simulink model "Simulador_Telemetria"  (R2015a)
settings: Solver=ode45  StartTime=0.0  StopTime=entrada2  RelTol=1e-6  AbsTol=1e-6
StopFcn:
  | close all;
  | post_simulacion_telemetria;
model workspace (MAT data in the model file):
  m = 3.797
  b = 2.1
  c = 0.3571
  Salar = 0.75
  AR = 5.88
  cg = [0.44 0 0]
  Ix = 1.229
  Iy = 0.1702
  Iz = 0.8808
  Ixz = 0.9343
  e = 0.9935
  alpha0 = 0.267
  coefprop = [0.016415 -0.0142726]
  C_L0 = 0.0254
  C_Lalpha = 4.0191
  C_Lq = 3.8954
  C_Ldelta_e = 0.5872
  C_D0 = 0.0102
  C_Dbeta1 = -2.0864e-07
  C_Dbeta2 = 0.0671
  C_Dq = 0
  C_Ddelta_e = 0.8461
  C_Y0 = 3.2049e-18
  C_Ybeta = -0.1949
  C_Yp = -0.1172
  C_Yr = 0.0959
  C_Ydelta_a = -0.0696
  C_l0 = 1.1518e-18
  C_lbeta = -0.0765
  C_lp = -0.4018
  C_lr = 0.025
  C_ldelta_a = 0.2987
  C_m0 = 0.018
  C_malpha = -0.2524
  C_mq = -1.3047
  C_mdelta_e = -0.4857
  C_n0 = -2.2667e-07
  C_nbeta = 0.0403
  C_np = -0.0247
  C_nr = -0.1252
  C_ndelta_a = 0.0076
  gamma = 0.20958671
  gamma1 = 8.64638926772
  gamma2 = 7.15127867602
  gamma3 = 4.20255654569
  gamma4 = 4.4578208227
  gamma5 = -2.04582843713
  gamma6 = 5.48942420682
  gamma7 = 10.3736620037
  gamma8 = 5.86392142899
  C_p0 = -1.01045424588e-06
  C_pbeta = -0.14184539659
  C_pp = -1.79869539438
  C_pr = -0.45305525336
  C_pdelta_a = 1.28918307845
  C_r0 = -1.3291750703e-06
  C_rbeta = -0.104707259349
  C_rp = -1.93599126586
  C_rr = -0.622717442342
  C_rdelta_a = 1.3761168826
  C_mp = -0.2168
undefined symbols (not defined in the file or in its folder): magnitude
libraries: aerolibconvert2 x9, aerolibfltsims x2, instrumentlib x1, aerolibatmos2 x1, aerolibgravity2 x1
settings Model: TunableVars=GNSS,Viento  TunableVarsStorageClass=Auto,Auto  TunableVarsTypeQualifier=,  Creator=Cecilia Ruiz Romero  LastModifiedBy=Cecilia Ruiz Romero
settings SolverCC: ZeroCrossControl=EnableAll
settings DataIOCC: ExternalInput=[t,u]  SaveOutput=off  TimeSaveName=tiempos

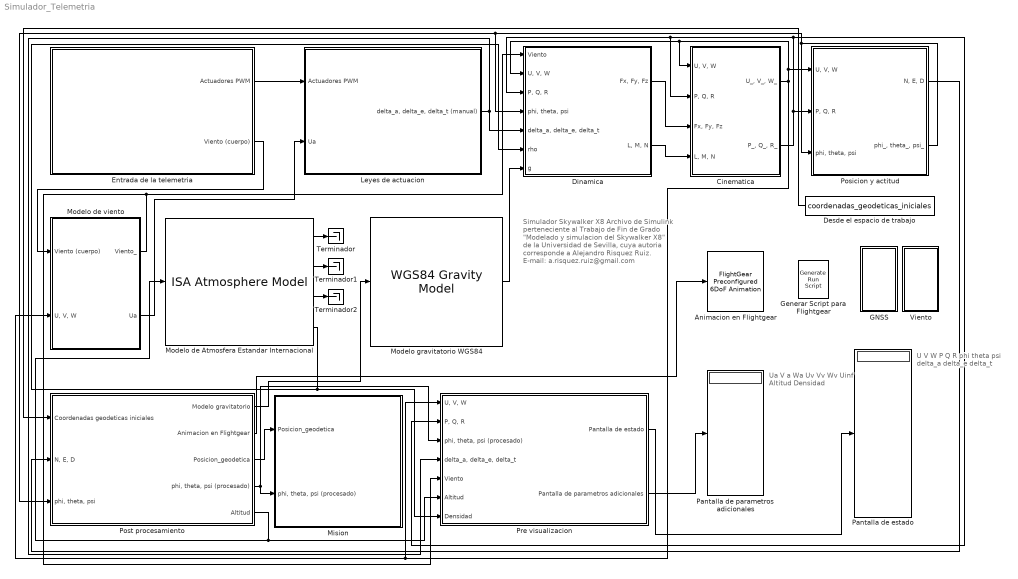
== system Simulador_Telemetria ==
  note: U
      | V
      | W
      | P
      | Q
      | R
      | phi
      | theta
      | psi
      | delta_a
      | delta_e
      | delta_t
  note: Ua
      | V a
      | Wa
      | Uv
      | Vv
      | Wv
      | Uinf
      | Altitud
      | Densidad
  note: Simulador Skywalker X8
      |
      | Archivo de Simulink perteneciente al Trabajo de Fin de Grado "Modelado y simulacion del Skywalker X8" de la Universidad de Sevilla, cuya autoria corresponde a Alejandro Risquez Ruiz.
      |
      | E-mail: a.risquez.ruiz@gmail.com
  Animacion en Flightgear : aerolibfltsims/FlightGear Preconfigured 6DoF Animation  xFlightGearVersion=v3.0  DestinationIpAddress=192.168.1.33  DestinationPort=5502  SampleTime=1/30
  Cinematica : Subsystem
  Desde el espacio de trabajo : FromWorkspace  VariableName=coordenadas_geodeticas_iniciales
  Dinamica : Subsystem
  Entrada de la telemetria : Subsystem
  GNSS : Subsystem  DialogController=hmiCreateDDGDialog  IsWebBlock=on  mask(MathWorksWebBlock){webBlockId=2f82c36a-ef1f-4a61-96ee-8f2028b7861b, webBlockType=toggleswitch, ShowInLibBrowser=on, ShowInitialText=on, HMISrcModelName=Simulador_Telemetria}
      mask prompts: webBlockId "WebBlock Id"; webBlockType "WebBlock Type"; HMISrcModelName "Source Model"
      mask Help: helpview([docroot '/mapfiles/simulink.map'], 'hmi_toggle_switch')
      mask Display:
      | if strcmp(get_param(bdroot(gcb),'BlockDiagramType'), 'library')
      |     image([(matlabroot) '/toolbox/simulink/hmi/icons/ToggleSwitch.png']);
      | end
  Generar Script para Flightgear : aerolibfltsims/Generate Run Script  OutputFileName=Flightgear_simulador.bat  FlightGearBaseDirectory=C:\Program Files\FlightGear  GeometryModelName=Malolo1  DestinationPort=5502  OriginAddress=192.168.1.34  OriginPort=5505  LocalAddress=192.168.1.35  AirportId=LEZL  RunwayId=27  InitialAltitude=328  InitialHeading=270  OffsetDistance=0  OffsetAzimuth=0  GenerateFile=off  Architecture=Win64  dataFlow=Receive
  Leyes de actuacion : Subsystem
  Mision : Subsystem
  Modelo de Atmosfera Estandar Internacional : aerolibatmos2/ISA Atmosphere Model  custom=off  g=9.80665  gamma=1.4  R=287.0531  L=0.0065  h_trop=11000  h_strat=20000  rho0=1.225  P0=101325  T0=288.15  h0=0
  Modelo de viento : Subsystem
  Modelo gravitatorio WGS84 : aerolibgravity2/WGS84 Gravity Model   model=WGS84 Taylor Series  units=Metric (MKS)  no_atmos=on  precessing=on  jd_loc=off  month=October  day=10  year=2004  no_centrifugal=on  action=Warning
  Pantalla de estado : Display
  Pantalla de parametros adicionales : Display
  Posicion y actitud : Subsystem
  Post procesamiento : Subsystem
  Pre visualizacion : Subsystem
  Terminador : Terminator
  Terminador1 : Terminator
  Terminador2 : Terminator
  Viento : Subsystem  DialogController=hmiCreateDDGDialog  IsWebBlock=on  mask(MathWorksWebBlock){webBlockId=de649073-e8b6-4552-a188-ccf5b7e05afd, webBlockType=toggleswitch, ShowInLibBrowser=on, ShowInitialText=on, HMISrcModelName=Simulador_Telemetria}
      mask prompts: webBlockId "WebBlock Id"; webBlockType "WebBlock Type"; HMISrcModelName "Source Model"
      mask Help: helpview([docroot '/mapfiles/simulink.map'], 'hmi_toggle_switch')
      mask Display:
      | if strcmp(get_param(bdroot(gcb),'BlockDiagramType'), 'library')
      |     image([(matlabroot) '/toolbox/simulink/hmi/icons/ToggleSwitch.png']);
      | end
  wires:
  Modelo de Atmosfera Estandar Internacional/1 -> Terminador/1
  Modelo de Atmosfera Estandar Internacional/2 -> Terminador1/1
  Modelo de Atmosfera Estandar Internacional/3 -> Terminador2/1
  Post procesamiento/5(Altitud) -> Modelo de Atmosfera Estandar Internacional/1, Pre visualizacion/6(Altitud)
  Cinematica/1("U_, V_, W_") -> Modelo de viento/2("U, V, W"), Pre visualizacion/1("U, V, W"), Dinamica/2("U, V, W"), Cinematica/1("U, V, W"), Posicion y actitud/1("U, V, W")
  Modelo de viento/1(Viento_) -> Pre visualizacion/5(Viento), Dinamica/1(Viento)
  Modelo de Atmosfera Estandar Internacional/4 -> Pre visualizacion/7(Densidad), Dinamica/6(rho)
  Cinematica/2("P_, Q_, R_") -> Dinamica/3("P, Q, R"), Cinematica/2("P, Q, R"), Pre visualizacion/2("P, Q, R"), Posicion y actitud/2("P, Q, R")
  Posicion y actitud/2("phi_, theta_, psi_") -> Posicion y actitud/3("phi, theta, psi"), Post procesamiento/3("phi, theta, psi"), Dinamica/4("phi, theta, psi")
  Dinamica/1("Fx, Fy, Fz") -> Cinematica/3("Fx, Fy, Fz")
  Dinamica/2("L, M, N") -> Cinematica/4("L, M, N")
  Posicion y actitud/1("N, E, D") -> Post procesamiento/2("N, E, D")
  Post procesamiento/2(Animacion en Flightgear) -> Animacion en Flightgear/1
  Post procesamiento/3(Posicion_geodetica) -> Mision/1(Posicion_geodetica)
  Post procesamiento/4("phi, theta, psi (procesado)") -> Mision/2("phi, theta, psi (procesado)"), Pre visualizacion/3("phi, theta, psi (procesado)")
  Pre visualizacion/1(Pantalla de estado) -> Pantalla de estado/1
  Pre visualizacion/2(Pantalla de parametros adicionales) -> Pantalla de parametros adicionales/1
  Modelo de viento/2(Ua) -> Leyes de actuacion/2(Ua)
  Modelo gravitatorio WGS84/1 -> Dinamica/7(g)
  Post procesamiento/1(Modelo gravitatorio) -> Modelo gravitatorio WGS84/1
  Leyes de actuacion/1("delta_a, delta_e, delta_t (manual)") -> Dinamica/5("delta_a, delta_e, delta_t"), Pre visualizacion/4("delta_a, delta_e, delta_t")
  Entrada de la telemetria/1(Actuadores PWM) -> Leyes de actuacion/1(Actuadores PWM)
  Entrada de la telemetria/2(Viento (cuerpo)) -> Modelo de viento/1(Viento (cuerpo))
  Desde el espacio de trabajo/1 -> Post procesamiento/1(Coordenadas geodeticas iniciales)

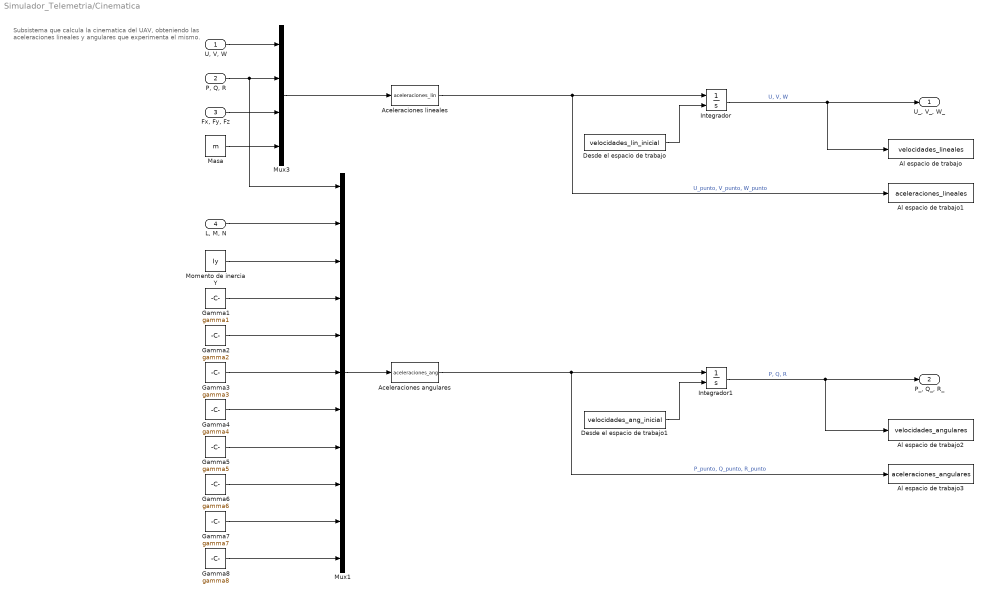
== system Simulador_Telemetria/Cinematica ==
  note: Subsistema que calcula la cinematica del
      | UAV, obteniendo las aceleraciones lineales
      | y angulares que experimenta el mismo.
  "U, V, W" : Inport
  "P, Q, R" : Inport  Port=2
  "Fx, Fy, Fz" : Inport  Port=3
  "L, M, N" : Inport  Port=4
  Aceleraciones angulares : MATLABFcn  MATLABFcn=aceleraciones_ang  OutputDimensions=3
  Aceleraciones lineales : MATLABFcn  MATLABFcn=aceleraciones_lin  OutputDimensions=3
  Al espacio de trabajo : ToWorkspace  VariableName=velocidades_lineales  SaveFormat=Timeseries  SampleTime=-1
  Al espacio de trabajo1 : ToWorkspace  VariableName=aceleraciones_lineales  SaveFormat=Timeseries  SampleTime=-1
  Al espacio de trabajo2 : ToWorkspace  VariableName=velocidades_angulares  SaveFormat=Timeseries  SampleTime=-1
  Al espacio de trabajo3 : ToWorkspace  VariableName=aceleraciones_angulares  SaveFormat=Timeseries  SampleTime=-1
  Desde el espacio de trabajo : FromWorkspace  VariableName=velocidades_lin_inicial
  Desde el espacio de trabajo1 : FromWorkspace  VariableName=velocidades_ang_inicial
  Gamma1 : Constant  Value=gamma1
  Gamma2 : Constant  Value=gamma2
  Gamma3 : Constant  Value=gamma3
  Gamma4 : Constant  Value=gamma4
  Gamma5 : Constant  Value=gamma5
  Gamma6 : Constant  Value=gamma6
  Gamma7 : Constant  Value=gamma7
  Gamma8 : Constant  Value=gamma8
  Integrador : Integrator  InitialConditionSource=external  InitialCondition=[22.5000 1.20777e-04 0.678706]
  Integrador1 : Integrator  InitialConditionSource=external  InitialCondition=[-6.87125e-22 -3.91163e-24 -2.13625e-23]
  Masa : Constant  Value=m
  Momento de inercia Y : Constant  Value=Iy
  Mux1 : Mux  Inputs=11
  Mux3 : Mux
  "U_, V_, W_" : Outport
  "P_, Q_, R_" : Outport  Port=2
  wires:
  Aceleraciones lineales/1 -> Integrador/1, Al espacio de trabajo1/1  "U_punto, V_punto, W_punto"
  Aceleraciones angulares/1 -> Integrador1/1, Al espacio de trabajo3/1  "P_punto, Q_punto, R_punto"
  "U, V, W"/1 -> Mux3/1
  "P, Q, R"/1 -> Mux3/2, Mux1/1
  "Fx, Fy, Fz"/1 -> Mux3/3
  "L, M, N"/1 -> Mux1/2
  Mux3/1 -> Aceleraciones lineales/1
  Mux1/1 -> Aceleraciones angulares/1
  Integrador/1 -> "U_, V_, W_"/1, Al espacio de trabajo/1  "U, V, W"
  Integrador1/1 -> "P_, Q_, R_"/1, Al espacio de trabajo2/1  "P, Q, R"
  Momento de inercia Y/1 -> Mux1/3
  Gamma1/1 -> Mux1/4
  Gamma2/1 -> Mux1/5
  Gamma3/1 -> Mux1/6
  Gamma4/1 -> Mux1/7
  Gamma5/1 -> Mux1/8
  Gamma6/1 -> Mux1/9
  Gamma7/1 -> Mux1/10
  Gamma8/1 -> Mux1/11
  Masa/1 -> Mux3/4
  Desde el espacio de trabajo/1 -> Integrador/2
  Desde el espacio de trabajo1/1 -> Integrador1/2

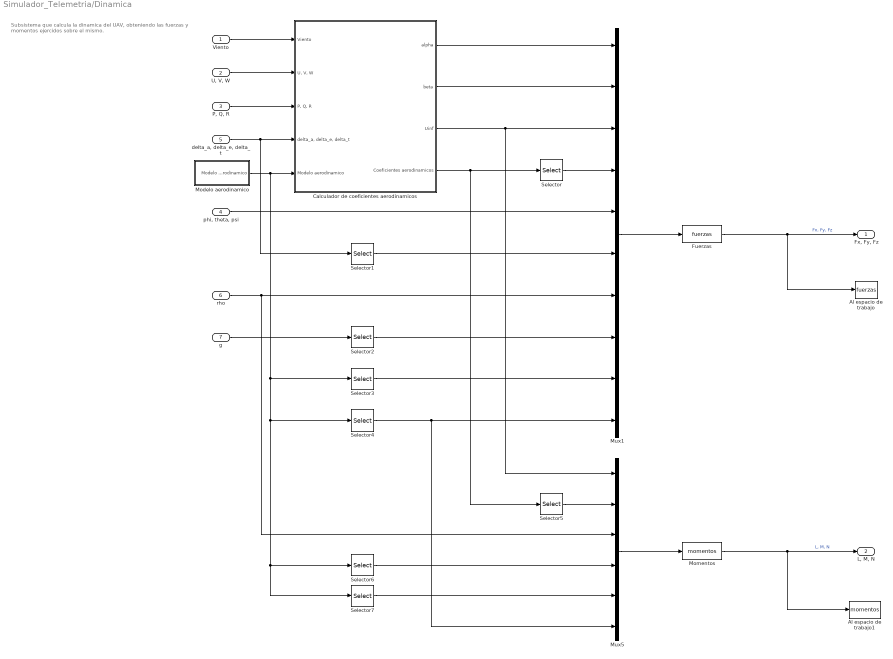
== system Simulador_Telemetria/Dinamica ==
  note: Subsistema que calcula la dinamica
      | del UAV, obteniendo las fuerzas y
      | momentos ejercidos sobre el mismo.
  Viento : Inport
  "U, V, W" : Inport  Port=2
  "P, Q, R" : Inport  Port=3
  "phi, theta, psi" : Inport  Port=4
  "delta_a, delta_e, delta_t" : Inport  Port=5
  rho : Inport  Port=6
  g : Inport  Port=7
  Al espacio de trabajo : ToWorkspace  VariableName=fuerzas  SaveFormat=Timeseries  SampleTime=-1
  Al espacio de trabajo1 : ToWorkspace  VariableName=momentos  SaveFormat=Timeseries  SampleTime=-1
  Calculador de coeficientes aerodinamicos : Subsystem
  Fuerzas : MATLABFcn  MATLABFcn=fuerzas  OutputDimensions=3
  Modelo aerodinamico : Subsystem
  Momentos : MATLABFcn  MATLABFcn=momentos  OutputDimensions=3
  Mux1 : Mux  Inputs=10
  Mux5 : Mux  Inputs=6
  Selector : Selector  InputPortWidth=6  Indices=[1 2 3]
  Selector1 : Selector  InputPortWidth=3  Indices=3
  Selector2 : Selector  InputPortWidth=3  Indices=3
  Selector3 : Selector  InputPortWidth=35
  Selector4 : Selector  InputPortWidth=35  Indices=4
  Selector5 : Selector  InputPortWidth=6  Indices=[4 5 6]
  Selector6 : Selector  InputPortWidth=35  Indices=2
  Selector7 : Selector  InputPortWidth=35  Indices=3
  "Fx, Fy, Fz" : Outport
  "L, M, N" : Outport  Port=2
  wires:
  Momentos/1 -> "L, M, N"/1, Al espacio de trabajo1/1  "L, M, N"
  g/1 -> Selector2/1
  "delta_a, delta_e, delta_t"/1 -> Selector1/1, Calculador de coeficientes aerodinamicos/4("delta_a, delta_e, delta_t")
  Viento/1 -> Calculador de coeficientes aerodinamicos/1(Viento)
  "U, V, W"/1 -> Calculador de coeficientes aerodinamicos/2("U, V, W")
  "P, Q, R"/1 -> Calculador de coeficientes aerodinamicos/3("P, Q, R")
  Calculador de coeficientes aerodinamicos/4(Coeficientes aerodinamicos) -> Selector/1, Selector5/1
  rho/1 -> Mux5/3, Mux1/7
  Mux1/1 -> Fuerzas/1
  Mux5/1 -> Momentos/1
  Modelo aerodinamico/1(Modelo aerodinamico) -> Selector7/1, Selector6/1, Selector4/1, Selector3/1, Calculador de coeficientes aerodinamicos/5(Modelo aerodinamico)
  Selector4/1 -> Mux5/6, Mux1/10
  Calculador de coeficientes aerodinamicos/1(alpha) -> Mux1/1
  Calculador de coeficientes aerodinamicos/2(beta) -> Mux1/2
  Selector/1 -> Mux1/4
  Calculador de coeficientes aerodinamicos/3(Uinf) -> Mux5/1, Mux1/3
  "phi, theta, psi"/1 -> Mux1/5
  Selector1/1 -> Mux1/6
  Selector2/1 -> Mux1/8
  Selector3/1 -> Mux1/9
  Selector7/1 -> Mux5/5
  Selector6/1 -> Mux5/4
  Selector5/1 -> Mux5/2
  Fuerzas/1 -> "Fx, Fy, Fz"/1, Al espacio de trabajo/1  "Fx, Fy, Fz"

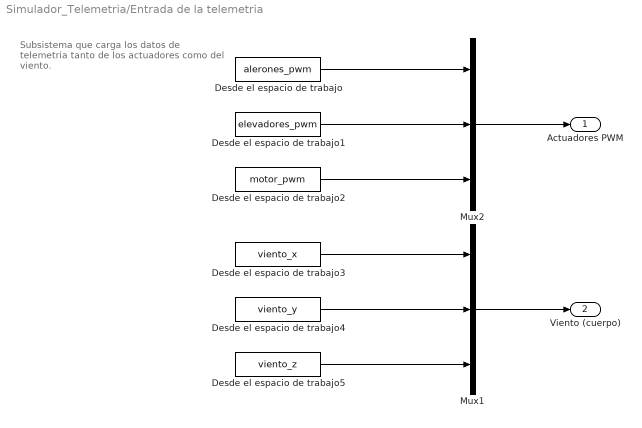
== system Simulador_Telemetria/Entrada de la telemetria ==
  note: Subsistema que carga los datos de telemetria
      | tanto de los actuadores como del viento.
  Desde el espacio de trabajo : FromWorkspace  VariableName=alerones_pwm
  Desde el espacio de trabajo1 : FromWorkspace  VariableName=elevadores_pwm
  Desde el espacio de trabajo2 : FromWorkspace  VariableName=motor_pwm
  Desde el espacio de trabajo3 : FromWorkspace  VariableName=viento_x
  Desde el espacio de trabajo4 : FromWorkspace  VariableName=viento_y
  Desde el espacio de trabajo5 : FromWorkspace  VariableName=viento_z
  Mux1 : Mux  Inputs=3
  Mux2 : Mux  Inputs=3
  Actuadores PWM : Outport
  Viento (cuerpo) : Outport  Port=2
  wires:
  Desde el espacio de trabajo3/1 -> Mux1/1
  Desde el espacio de trabajo4/1 -> Mux1/2
  Desde el espacio de trabajo5/1 -> Mux1/3
  Mux1/1 -> Viento (cuerpo)/1
  Mux2/1 -> Actuadores PWM/1
  Desde el espacio de trabajo2/1 -> Mux2/3
  Desde el espacio de trabajo/1 -> Mux2/1
  Desde el espacio de trabajo1/1 -> Mux2/2

== system Simulador_Telemetria/GNSS ==

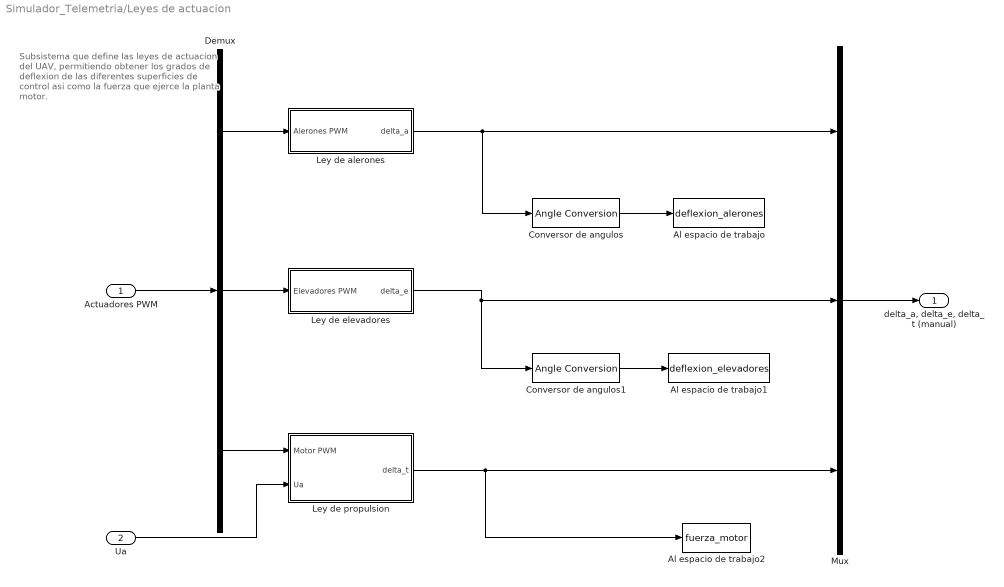
== system Simulador_Telemetria/Leyes de actuacion ==
  note: Subsistema que define las leyes de actuacion
      | del UAV, permitiendo obtener los grados de
      | deflexion de las diferentes superficies de control
      | asi como la fuerza que ejerce la planta motor.
  Actuadores PWM : Inport
  Ua : Inport  Port=2
  Al espacio de trabajo : ToWorkspace  VariableName=deflexion_alerones  SaveFormat=Timeseries  SampleTime=-1
  Al espacio de trabajo1 : ToWorkspace  VariableName=deflexion_elevadores  SaveFormat=Timeseries  SampleTime=-1
  Al espacio de trabajo2 : ToWorkspace  VariableName=fuerza_motor  SaveFormat=Timeseries  SampleTime=-1
  Conversor de angulos : aerolibconvert2/Angle Conversion  IU=rad  OU=deg
  Conversor de angulos1 : aerolibconvert2/Angle Conversion  IU=rad  OU=deg
  Demux : Demux  Outputs=3
  Ley de alerones : Subsystem
  Ley de elevadores : Subsystem
  Ley de propulsion : Subsystem
  Mux : Mux  Inputs=3
  "delta_a, delta_e, delta_t (manual)" : Outport
  wires:
  Ley de propulsion/1(delta_t) -> Al espacio de trabajo2/1, Mux/3
  Ua/1 -> Ley de propulsion/2(Ua)
  Ley de alerones/1(delta_a) -> Conversor de angulos/1, Mux/1
  Ley de elevadores/1(delta_e) -> Conversor de angulos1/1, Mux/2
  Conversor de angulos/1 -> Al espacio de trabajo/1
  Conversor de angulos1/1 -> Al espacio de trabajo1/1
  Demux/2 -> Ley de elevadores/1(Elevadores PWM)
  Demux/3 -> Ley de propulsion/1(Motor PWM)
  Demux/1 -> Ley de alerones/1(Alerones PWM)
  Actuadores PWM/1 -> Demux/1
  Mux/1 -> "delta_a, delta_e, delta_t (manual)"/1

== system Simulador_Telemetria/Mision ==
  note: Subsistema que desarrolla la logica del bloque
      | de mision, incluyendo un sistema de gestion
      | del vuelo asi como un receptor de un
      | sistema de posicionamiento por satelite.
  Posicion_geodetica : Inport  SampleTime=1
  "phi, theta, psi (procesado)" : Inport  Port=2  SampleTime=1
  Al espacio de trabajo : ToWorkspace  VariableName=posicion_geodetica  SaveFormat=Timeseries  SampleTime=-1
  Conversor de angulos : aerolibconvert2/Angle Conversion  IU=rad  OU=deg
  GNSS : Constant  Value=0
  Gestor de GPS : Subsystem
  Selector : Selector  InputPortWidth=3  Indices=3
  wires:
  "phi, theta, psi (procesado)"/1 -> Conversor de angulos/1
  GNSS/1 -> Gestor de GPS/Enable
  Conversor de angulos/1 -> Selector/1
  Selector/1 -> Gestor de GPS/2("Psi ")
  Posicion_geodetica/1 -> Al espacio de trabajo/1, Gestor de GPS/1(Posicion_geodetica)

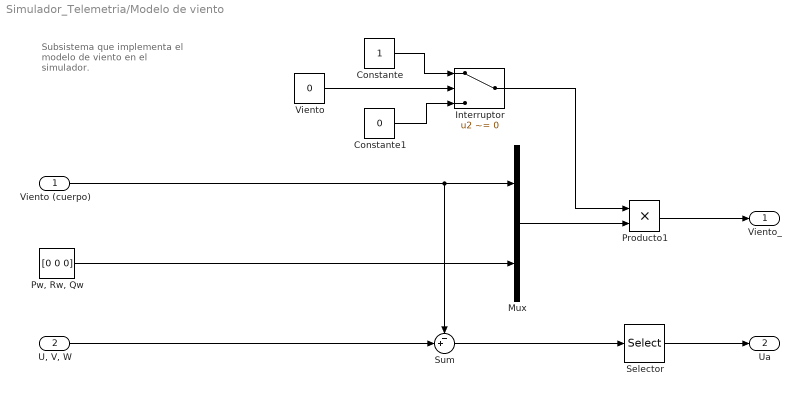
== system Simulador_Telemetria/Modelo de viento ==
  note: Subsistema que implementa el
      | modelo de viento en el simulador.
  Viento (cuerpo) : Inport
  "U, V, W" : Inport  Port=2
  Constante : Constant
  Constante1 : Constant  Value=0
  Interruptor : Switch  Criteria=u2 ~= 0
  Mux : Mux  Inputs=2
  Producto1 : Product
  "Pw, Rw, Qw" : Constant  Value=[0 0 0]
  Selector : Selector  InputPortWidth=3
  Sum : Sum  Inputs=-+|
  Viento : Constant  Value=0  OutDataTypeStr=boolean
  Viento_ : Outport
  Ua : Outport  Port=2
  wires:
  Viento/1 -> Interruptor/2
  "U, V, W"/1 -> Sum/2
  Selector/1 -> Ua/1
  Sum/1 -> Selector/1
  Interruptor/1 -> Producto1/1
  Constante/1 -> Interruptor/1
  Constante1/1 -> Interruptor/3
  "Pw, Rw, Qw"/1 -> Mux/2
  Mux/1 -> Producto1/2
  Producto1/1 -> Viento_/1
  Viento (cuerpo)/1 -> Sum/1, Mux/1

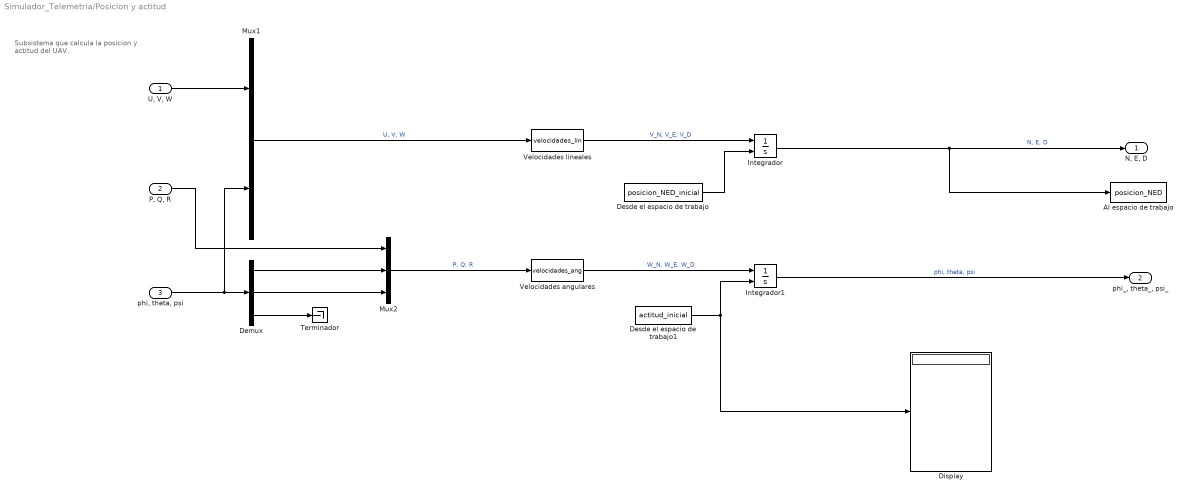
== system Simulador_Telemetria/Posicion y actitud ==
  note: Subsistema que calcula la
      | posicion y actitud del UAV.
  "U, V, W" : Inport
  "P, Q, R" : Inport  Port=2
  "phi, theta, psi" : Inport  Port=3
  Al espacio de trabajo : ToWorkspace  VariableName=posicion_NED  SaveFormat=Timeseries  SampleTime=-1
  Demux : Demux  Outputs=3
  Desde el espacio de trabajo : FromWorkspace  VariableName=posicion_NED_inicial
  Desde el espacio de trabajo1 : FromWorkspace  VariableName=actitud_inicial
  Display : Display
  Integrador : Integrator  InitialConditionSource=external  InitialCondition=[0 0 0]
  Integrador1 : Integrator  InitialConditionSource=external  InitialCondition=[8.12415e-06 0.0301555 270*pi/180]
  Mux1 : Mux  Inputs=2
  Mux2 : Mux  Inputs=3
  Terminador : Terminator
  Velocidades angulares : MATLABFcn  MATLABFcn=velocidades_ang  OutputDimensions=3
  Velocidades lineales : MATLABFcn  MATLABFcn=velocidades_lin  OutputDimensions=3
  "N, E, D" : Outport
  "phi_, theta_, psi_" : Outport  Port=2
  wires:
  Velocidades lineales/1 -> Integrador/1  "V_N, V_E, V_D"
  Velocidades angulares/1 -> Integrador1/1  "W_N, W_E, W_D"
  Mux1/1 -> Velocidades lineales/1  "U, V, W"
  "phi, theta, psi"/1 -> Demux/1, Mux1/2
  Demux/1 -> Mux2/2
  Demux/2 -> Mux2/3
  Mux2/1 -> Velocidades angulares/1  "P, Q, R"
  Demux/3 -> Terminador/1
  Integrador/1 -> "N, E, D"/1, Al espacio de trabajo/1  "N, E, D"
  "P, Q, R"/1 -> Mux2/1
  Integrador1/1 -> "phi_, theta_, psi_"/1  "phi, theta, psi"
  "U, V, W"/1 -> Mux1/1
  Desde el espacio de trabajo/1 -> Integrador/2
  Desde el espacio de trabajo1/1 -> Integrador1/2, Display/1

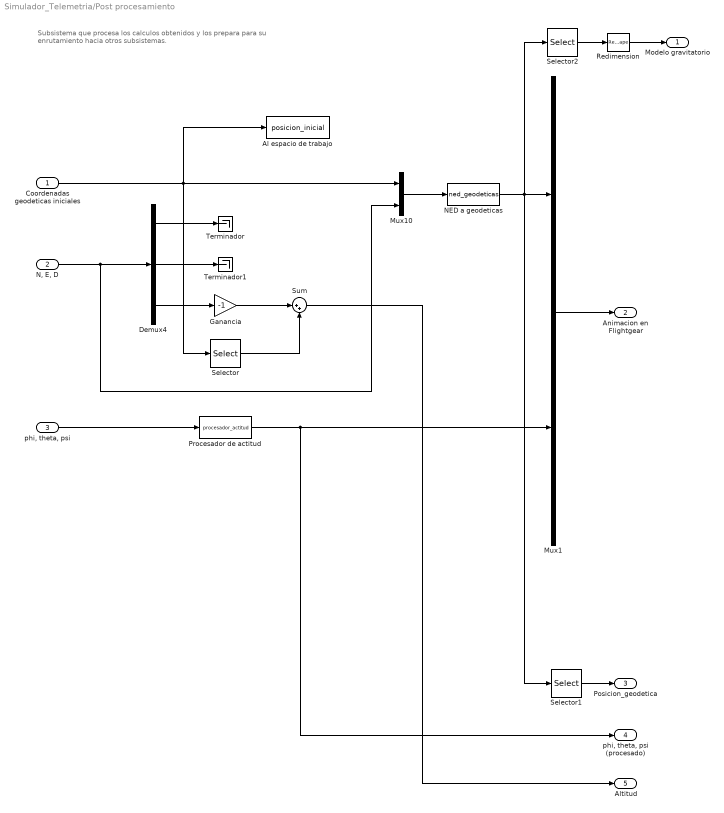
== system Simulador_Telemetria/Post procesamiento ==
  note: Subsistema que procesa los calculos
      | obtenidos y los prepara para su
      | enrutamiento hacia otros subsistemas.
  Coordenadas geodeticas iniciales : Inport
  "N, E, D" : Inport  Port=2
  "phi, theta, psi" : Inport  Port=3
  Al espacio de trabajo : ToWorkspace  VariableName=posicion_inicial  SaveFormat=Timeseries  SampleTime=-1
  Demux4 : Demux  Outputs=3
  Ganancia : Gain  Gain=-1
  Mux1 : Mux  Inputs=2
  Mux10 : Mux  Inputs=2
  NED a geodeticas : MATLABFcn  MATLABFcn=ned_geodeticas  OutputDimensions=3
  Procesador de actitud : MATLABFcn  MATLABFcn=procesador_actitud  OutputDimensions=3
  Redimension : Reshape
  Selector : Selector  InputPortWidth=3  Indices=3
  Selector1 : Selector  InputPortWidth=3  Indices=[2 1 3]
  Selector2 : Selector  InputPortWidth=3  Indices=[2 1 3]
  Sum : Sum  Inputs=|++
  Terminador : Terminator
  Terminador1 : Terminator
  Modelo gravitatorio : Outport
  Animacion en Flightgear : Outport  Port=2
  Posicion_geodetica : Outport  Port=3
  "phi, theta, psi (procesado)" : Outport  Port=4
  Altitud : Outport  Port=5
  wires:
  Demux4/1 -> Terminador/1
  Demux4/2 -> Terminador1/1
  Demux4/3 -> Ganancia/1
  Ganancia/1 -> Sum/1
  Selector/1 -> Sum/2
  "N, E, D"/1 -> Mux10/2, Demux4/1
  Mux10/1 -> NED a geodeticas/1
  NED a geodeticas/1 -> Selector2/1, Selector1/1, Mux1/1
  Mux1/1 -> Animacion en Flightgear/1
  Selector1/1 -> Posicion_geodetica/1
  Procesador de actitud/1 -> "phi, theta, psi (procesado)"/1, Mux1/2
  "phi, theta, psi"/1 -> Procesador de actitud/1
  Sum/1 -> Altitud/1
  Selector2/1 -> Redimension/1
  Redimension/1 -> Modelo gravitatorio/1
  Coordenadas geodeticas iniciales/1 -> Al espacio de trabajo/1, Selector/1, Mux10/1

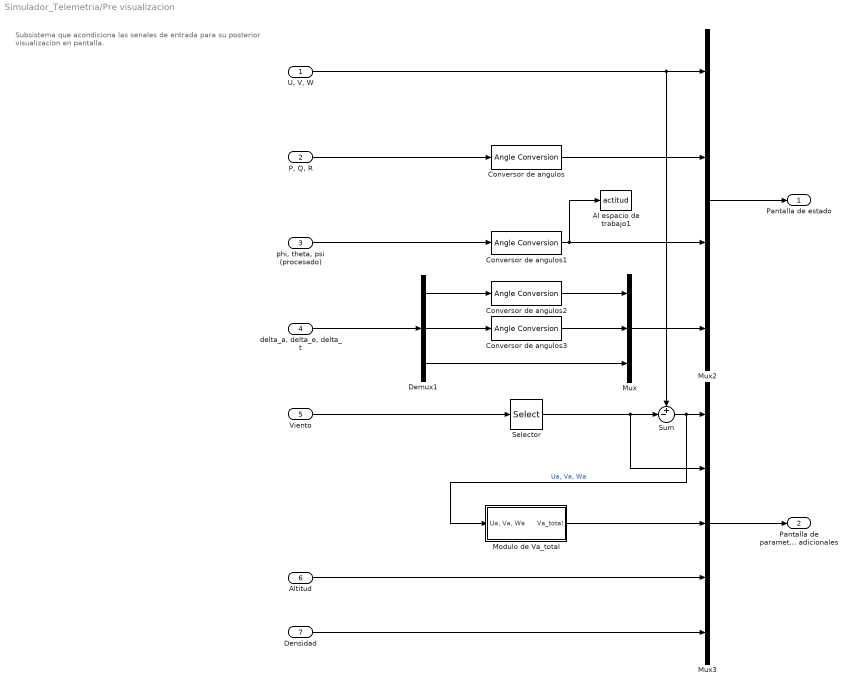
== system Simulador_Telemetria/Pre visualizacion ==
  note: Subsistema que acondiciona las
      | senales de entrada para su posterior
      | visualizacion en pantalla.
  "U, V, W" : Inport
  "P, Q, R" : Inport  Port=2
  "phi, theta, psi (procesado)" : Inport  Port=3
  "delta_a, delta_e, delta_t" : Inport  Port=4
  Viento : Inport  Port=5
  Altitud : Inport  Port=6
  Densidad : Inport  Port=7
  Al espacio de trabajo1 : ToWorkspace  VariableName=actitud  SaveFormat=Timeseries  SampleTime=-1
  Conversor de angulos{,1..3} (4 alike) : aerolibconvert2/Angle Conversion  IU=rad  OU=deg
  Demux1 : Demux  Outputs=3
  Modulo de Va_total : Subsystem
  Mux : Mux  Inputs=3
  Mux2 : Mux
  Mux3 : Mux  Inputs=5
  Selector : Selector  InputPortWidth=6  Indices=[1 2 3]
  Sum : Sum  Inputs=+-|
  Pantalla de estado : Outport
  Pantalla de parametros adicionales : Outport  Port=2
  wires:
  Conversor de angulos2/1 -> Mux/1
  Conversor de angulos3/1 -> Mux/2
  Demux1/2 -> Conversor de angulos3/1
  Demux1/1 -> Conversor de angulos2/1
  Demux1/3 -> Mux/3
  Mux/1 -> Mux2/4
  Mux2/1 -> Pantalla de estado/1
  "delta_a, delta_e, delta_t"/1 -> Demux1/1
  "phi, theta, psi (procesado)"/1 -> Conversor de angulos1/1
  "U, V, W"/1 -> Mux2/1, Sum/1
  Conversor de angulos/1 -> Mux2/2
  "P, Q, R"/1 -> Conversor de angulos/1
  Viento/1 -> Selector/1
  Sum/1 -> Modulo de Va_total/1("Ua, Va, Wa"), Mux3/1  "Ua, Va, Wa"
  Mux3/1 -> Pantalla de parametros adicionales/1
  Selector/1 -> Mux3/2, Sum/2
  Conversor de angulos1/1 -> Mux2/3, Al espacio de trabajo1/1
  Densidad/1 -> Mux3/5
  Altitud/1 -> Mux3/4
  Modulo de Va_total/1(Va_total) -> Mux3/3

== system Simulador_Telemetria/Viento ==

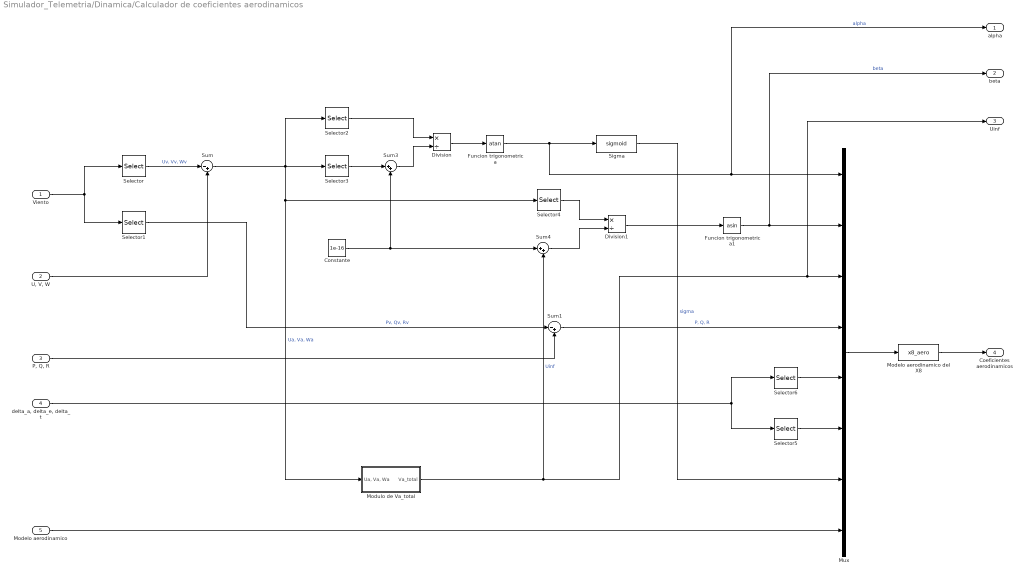
== system Simulador_Telemetria/Dinamica/Calculador de coeficientes aerodinamicos ==
  Viento : Inport
  "U, V, W" : Inport  Port=2
  "P, Q, R" : Inport  Port=3
  "delta_a, delta_e, delta_t" : Inport  Port=4
  Modelo aerodinamico : Inport  Port=5
  Constante : Constant  Value=1e-16
  Division : Product  Inputs=*/
  Division1 : Product  Inputs=*/
  Funcion trigonometrica : Trigonometry  Operator=atan
  Funcion trigonometrica1 : Trigonometry  Operator=asin
  Modelo aerodinamico del X8 : MATLABFcn  MATLABFcn=x8_aero  OutputDimensions=6
  Modulo de Va_total : Subsystem
  Mux : Mux  Inputs=8
  Selector : Selector  InputPortWidth=6  Indices=[1 2 3]
  Selector1 : Selector  InputPortWidth=6  Indices=[4 5 6]
  Selector2 : Selector  InputPortWidth=3  Indices=3
  Selector3 : Selector  InputPortWidth=3
  Selector4 : Selector  InputPortWidth=3  Indices=2
  Selector5 : Selector  InputPortWidth=3  Indices=2
  Selector6 : Selector  InputPortWidth=3
  Sigma : MATLABFcn  MATLABFcn=sigmoid  OutputDimensions=1
  Sum : Sum  Inputs=|-+
  Sum1 : Sum  Inputs=|-+
  Sum3 : Sum  Inputs=|++
  Sum4 : Sum  Inputs=|++
  alpha : Outport
  beta : Outport  Port=2
  Uinf : Outport  Port=3
  Coeficientes aerodinamicos : Outport  Port=4
  wires:
  Viento/1 -> Selector/1, Selector1/1
  "U, V, W"/1 -> Sum/2
  Selector/1 -> Sum/1  "Uv, Vv, Wv"
  Selector1/1 -> Sum1/1  "Pv, Qv, Rv"
  "P, Q, R"/1 -> Sum1/2
  Sum/1 -> Selector3/1, Selector2/1, Selector4/1, Modulo de Va_total/1("Ua, Va, Wa")  "Ua, Va, Wa"
  Selector2/1 -> Division/1
  Sum3/1 -> Division/2
  Division/1 -> Funcion trigonometrica/1
  Division1/1 -> Funcion trigonometrica1/1
  Selector4/1 -> Division1/1
  Sum4/1 -> Division1/2
  Modulo de Va_total/1(Va_total) -> Uinf/1, Mux/3, Sum4/2  "Uinf"
  Funcion trigonometrica/1 -> Sigma/1, alpha/1, Mux/1  "alpha"
  Funcion trigonometrica1/1 -> Mux/2, beta/1  "beta"
  "delta_a, delta_e, delta_t"/1 -> Selector5/1, Selector6/1
  Mux/1 -> Modelo aerodinamico del X8/1
  Modelo aerodinamico del X8/1 -> Coeficientes aerodinamicos/1
  Constante/1 -> Sum4/1, Sum3/2
  Selector3/1 -> Sum3/1
  Sum1/1 -> Mux/4  "P, Q, R"
  Selector5/1 -> Mux/6
  Selector6/1 -> Mux/5
  Sigma/1 -> Mux/7  "sigma"
  Modelo aerodinamico/1 -> Mux/8

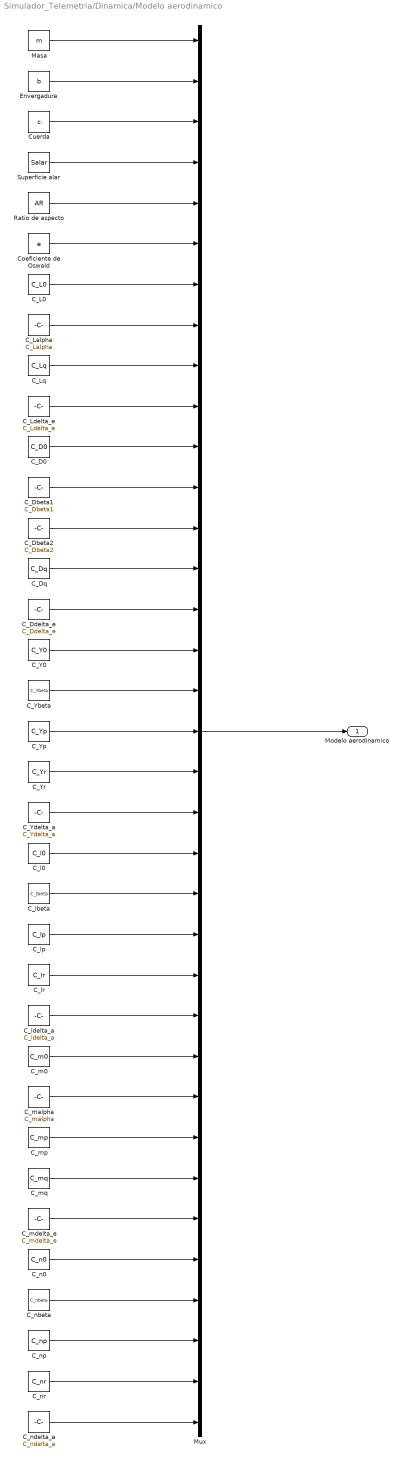
== system Simulador_Telemetria/Dinamica/Modelo aerodinamico ==
  C_D0 : Constant  Value=C_D0
  C_Dbeta1 : Constant  Value=C_Dbeta1
  C_Dbeta2 : Constant  Value=C_Dbeta2
  C_Ddelta_e : Constant  Value=C_Ddelta_e
  C_Dq : Constant  Value=C_Dq
  C_L0 : Constant  Value=C_L0
  C_Lalpha : Constant  Value=C_Lalpha
  C_Ldelta_e : Constant  Value=C_Ldelta_e
  C_Lq : Constant  Value=C_Lq
  C_Y0 : Constant  Value=C_Y0
  C_Ybeta : Constant  Value=C_Ybeta
  C_Ydelta_a : Constant  Value=C_Ydelta_a
  C_Yp : Constant  Value=C_Yp
  C_Yr : Constant  Value=C_Yr
  C_l0 : Constant  Value=C_l0
  C_lbeta : Constant  Value=C_lbeta
  C_ldelta_a : Constant  Value=C_ldelta_a
  C_lp : Constant  Value=C_lp
  C_lr : Constant  Value=C_lr
  C_m0 : Constant  Value=C_m0
  C_malpha : Constant  Value=C_malpha
  C_mdelta_e : Constant  Value=C_mdelta_e
  C_mp : Constant  Value=C_mp
  C_mq : Constant  Value=C_mq
  C_n0 : Constant  Value=C_n0
  C_nbeta : Constant  Value=C_nbeta
  C_ndelta_a : Constant  Value=C_ndelta_a
  C_np : Constant  Value=C_np
  C_nr : Constant  Value=C_nr
  Coeficiente de Oswald : Constant  Value=e
  Cuerda : Constant  Value=c
  Envergadura : Constant  Value=b
  Masa : Constant  Value=m
  Mux : Mux  Inputs=35
  Ratio de aspecto : Constant  Value=AR
  Superficie alar : Constant  Value=Salar
  Modelo aerodinamico : Outport
  wires:
  Mux/1 -> Modelo aerodinamico/1
  C_ndelta_a/1 -> Mux/35
  C_nr/1 -> Mux/34
  C_np/1 -> Mux/33
  C_nbeta/1 -> Mux/32
  C_n0/1 -> Mux/31
  C_mdelta_e/1 -> Mux/30
  C_mq/1 -> Mux/29
  C_mp/1 -> Mux/28
  C_malpha/1 -> Mux/27
  C_m0/1 -> Mux/26
  C_ldelta_a/1 -> Mux/25
  C_lr/1 -> Mux/24
  C_lp/1 -> Mux/23
  C_lbeta/1 -> Mux/22
  C_l0/1 -> Mux/21
  C_Ydelta_a/1 -> Mux/20
  C_Yr/1 -> Mux/19
  C_Yp/1 -> Mux/18
  C_Ybeta/1 -> Mux/17
  C_Y0/1 -> Mux/16
  C_Ddelta_e/1 -> Mux/15
  C_Dq/1 -> Mux/14
  C_Dbeta2/1 -> Mux/13
  C_Dbeta1/1 -> Mux/12
  C_D0/1 -> Mux/11
  C_Ldelta_e/1 -> Mux/10
  C_Lq/1 -> Mux/9
  C_Lalpha/1 -> Mux/8
  C_L0/1 -> Mux/7
  Masa/1 -> Mux/1
  Envergadura/1 -> Mux/2
  Cuerda/1 -> Mux/3
  Superficie alar/1 -> Mux/4
  Ratio de aspecto/1 -> Mux/5
  Coeficiente de Oswald/1 -> Mux/6

== system Simulador_Telemetria/Leyes de actuacion/Ley de alerones ==
  Alerones PWM : Inport
  Constante : Constant  Value=2*(2100-1520)
  Conversor de angulos : aerolibconvert2/Angle Conversion  IU=deg  OU=rad
  Division : Product  Inputs=*/
  PWM_0 : Constant  Value=1520
  Rango angular : Gain  Gain=10
  Saturacion : Saturate  UpperLimit=5  LowerLimit=-5
  Sum1 : Sum  Inputs=|+-
  delta_a : Outport
  wires:
  Alerones PWM/1 -> Sum1/1
  PWM_0/1 -> Sum1/2
  Sum1/1 -> Rango angular/1
  Rango angular/1 -> Division/1
  Constante/1 -> Division/2
  Division/1 -> Saturacion/1
  Conversor de angulos/1 -> delta_a/1
  Saturacion/1 -> Conversor de angulos/1

== system Simulador_Telemetria/Leyes de actuacion/Ley de elevadores ==
  Elevadores PWM : Inport
  Constante : Constant  Value=2*(2100-1520)
  Conversor de angulos : aerolibconvert2/Angle Conversion  IU=deg  OU=rad
  Division : Product  Inputs=*/
  Inversion : Gain  Gain=-1
  PWM_0 : Constant  Value=1520
  Rango angular : Gain  Gain=30
  Saturacion : Saturate  UpperLimit=15  LowerLimit=-15
  Sum1 : Sum  Inputs=|+-
  delta_e : Outport
  wires:
  PWM_0/1 -> Sum1/2
  Sum1/1 -> Rango angular/1
  Rango angular/1 -> Division/1
  Constante/1 -> Division/2
  Conversor de angulos/1 -> delta_e/1
  Saturacion/1 -> Conversor de angulos/1
  Elevadores PWM/1 -> Sum1/1
  Division/1 -> Inversion/1
  Inversion/1 -> Saturacion/1

== system Simulador_Telemetria/Leyes de actuacion/Ley de propulsion ==
  Motor PWM : Inport
  Ua : Inport  Port=2
  Coefprop_U^2 : Gain  Gain=coefprop(2)
  Coefprop_motor_pwm : Gain  Gain=coefprop(1)
  PWM_1 : Constant  Value=1100
  Producto : Product  Inputs=**
  Sum : Sum
  Sum1 : Sum  Inputs=|+-
  delta_t : Outport
  wires:
  Ua/1 -> Producto/2, Producto/1
  Motor PWM/1 -> Sum1/1
  PWM_1/1 -> Sum1/2
  Sum1/1 -> Coefprop_motor_pwm/1
  Producto/1 -> Coefprop_U^2/1
  Sum/1 -> delta_t/1
  Coefprop_U^2/1 -> Sum/2
  Coefprop_motor_pwm/1 -> Sum/1

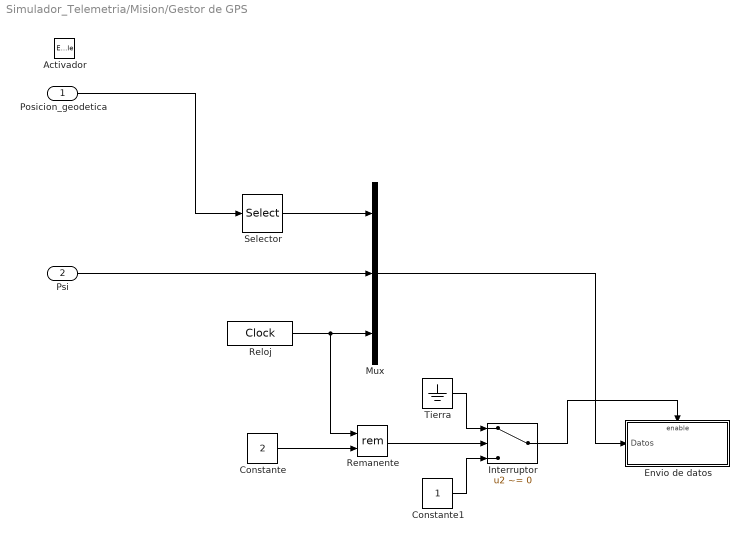
== system Simulador_Telemetria/Mision/Gestor de GPS ==
  Posicion_geodetica : Inport
  "Psi " : Inport  Port=2  SampleTime=1
  Activador : EnablePort
  Constante : Constant  Value=2
  Constante1 : Constant
  Envio de datos : Subsystem  TreatAsAtomicUnit=on
  Interruptor : Switch  Criteria=u2 ~= 0
  Mux : Mux  Inputs=3
  Reloj : DigitalClock
  Remanente : Math  Operator=rem  SaturateOnIntegerOverflow=on
  Selector : Selector  InputPortWidth=3  Indices=[1 2]
  Tierra : Ground
  wires:
  Reloj/1 -> Mux/3, Remanente/1
  Selector/1 -> Mux/1
  Constante/1 -> Remanente/2
  Remanente/1 -> Interruptor/2
  Constante1/1 -> Interruptor/3
  Tierra/1 -> Interruptor/1
  Interruptor/1 -> Envio de datos/Enable
  Mux/1 -> Envio de datos/1(Datos)
  "Psi "/1 -> Mux/2
  Posicion_geodetica/1 -> Selector/1

== system Simulador_Telemetria/Pre visualizacion/Modulo de Va_total ==
  "Ua, Va, Wa" : Inport
  Al cuadrado : Math  Operator=magnitude^2  SaturateOnIntegerOverflow=on
  Al cuadrado1 : Math  Operator=magnitude^2  SaturateOnIntegerOverflow=on
  Al cuadrado2 : Math  Operator=magnitude^2  SaturateOnIntegerOverflow=on
  Demux1 : Demux  Outputs=3
  Raiz cuadrada : Sqrt  SaturateOnIntegerOverflow=on
  Sum2 : Sum  Inputs=+++
  Va_total : Outport
  wires:
  "Ua, Va, Wa"/1 -> Demux1/1
  Demux1/2 -> Al cuadrado1/1
  Demux1/1 -> Al cuadrado/1
  Demux1/3 -> Al cuadrado2/1
  Al cuadrado1/1 -> Sum2/2
  Al cuadrado2/1 -> Sum2/3
  Al cuadrado/1 -> Sum2/1
  Sum2/1 -> Raiz cuadrada/1
  Raiz cuadrada/1 -> Va_total/1

== system Simulador_Telemetria/Dinamica/Calculador de coeficientes aerodinamicos/Modulo de Va_total ==
  "Ua, Va, Wa" : Inport
  Al cuadrado : Math  Operator=magnitude^2  SaturateOnIntegerOverflow=on
  Al cuadrado1 : Math  Operator=magnitude^2  SaturateOnIntegerOverflow=on
  Al cuadrado2 : Math  Operator=magnitude^2  SaturateOnIntegerOverflow=on
  Demux1 : Demux  Outputs=3
  Raiz cuadrada : Sqrt  SaturateOnIntegerOverflow=on
  Sum2 : Sum  Inputs=+++
  Va_total : Outport
  wires:
  "Ua, Va, Wa"/1 -> Demux1/1
  Demux1/2 -> Al cuadrado1/1
  Demux1/1 -> Al cuadrado/1
  Demux1/3 -> Al cuadrado2/1
  Al cuadrado1/1 -> Sum2/2
  Al cuadrado2/1 -> Sum2/3
  Al cuadrado/1 -> Sum2/1
  Sum2/1 -> Raiz cuadrada/1
  Raiz cuadrada/1 -> Va_total/1

== system Simulador_Telemetria/Mision/Gestor de GPS/Envio de datos ==
  Datos : Inport
  Activador : EnablePort
  Envio mediante protocolo UDP : instrumentlib/UDP Send  Host=localhost  Port=3333  LocalPort=3334  EnableBlockingMode=on  ByteOrder=BigEndian
  wires:
  Datos/1 -> Envio mediante protocolo UDP/1
